simulink subsystem "lift_compoenent"  (R2024b)
settings: Solver=VariableStepAuto  StartTime=0.0  StopTime=10.0  RelTol=1e-3
values from neighbouring files (symbols this model uses):
  Ar = 0.0181458391671    [barrowaman.mat]
  Lr = 0.152    [barrowaman.mat]
  OR_cg = [-2.50212 -2.5027 -2.50328 -2.50413 -2.50497 -2.50551 -2.50605 -2.50659 -2.5076 -2.5086 -2.50952 -2.51044 ... (1300 elements, 1300x1)]    [barrowaman.mat]
  sim_time = [0.01 0.02 0.03 0.04 0.05 0.06 0.07 0.08 0.09 0.1 0.11 0.12 ... (1300 elements, 1300x1)]    [barrowaman.mat]
libraries: sharedutil x2
settings Model: Creator=joedo  LastModifiedBy=joedo

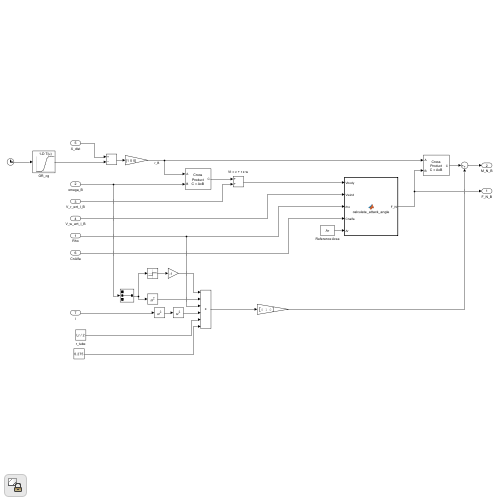
[thumbnail: Simulink's stored preview of the top-level diagram]
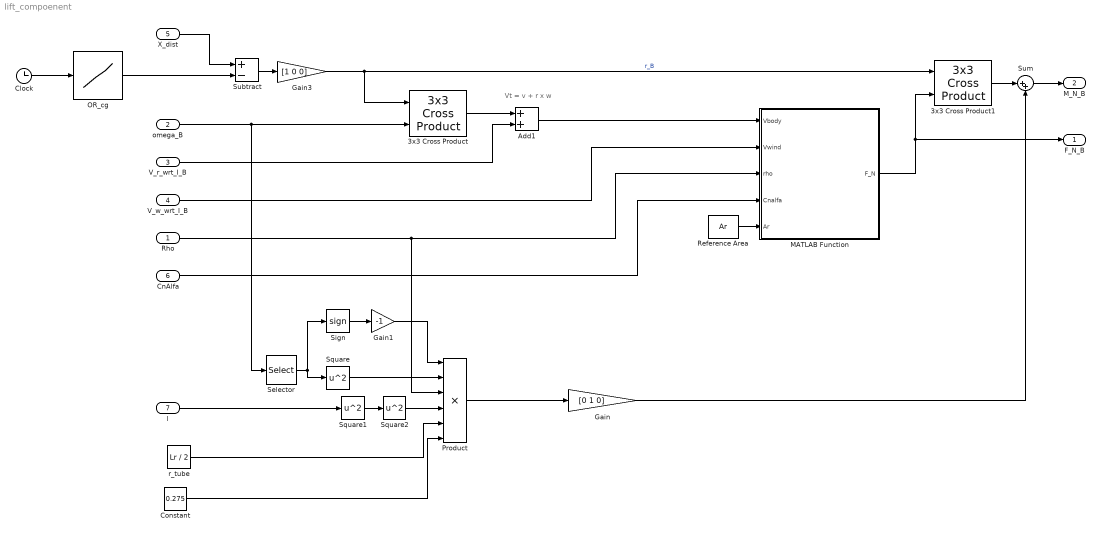
== system lift_compoenent ==
  note: Vt = v + r x w
  Rho : Inport
  omega_B : Inport  Port=2
  "V_r_wrt_I_B " : Inport  Port=3
  "V_w_wrt_I_B " : Inport  Port=4
  X_dist : Inport  Port=5
  CnAlfa : Inport  Port=6
  l : Inport  Port=7
  3x3 Cross Product : sharedutil/3x3 Cross Product  aMode=aMode
  3x3 Cross Product1 : sharedutil/3x3 Cross Product  aMode=aMode
  Add1 : Sum
  Clock : Clock
  Constant : Constant  Value=0.275
  Gain : Gain  Gain=[0 1 0]
  Gain1 : Gain  Gain=-1
  Gain3 : Gain  Gain=[1 0 0]
  MATLAB Function : MATLAB Function  TreatAsAtomicUnit=on
  OR_cg : Lookup_n-D  NumberOfTableDimensions=1  BreakpointsForDimension1=sim_time  Table=OR_cg  InternalRulePriority=Speed  RndMeth=Simplest
  Product : Product  Inputs=6
  Reference Area : Constant  Value=Ar
  Selector : Selector  InputPortWidth=3  IndexOptions=Index vector (dialog)  Indices=[2]  OutputSizes=1
  Sign : Signum
  Square : Math  Operator=square
  Square1 : Math  Operator=square
  Square2 : Math  Operator=square
  Subtract : Sum  Inputs=+-
  Sum : Sum  Inputs=|++
  r_tube : Constant  Value=Lr / 2
  F_N_B : Outport  VectorParamsAs1DForOutWhenUnconnected=off
  M_N_B : Outport  Port=2  VectorParamsAs1DForOutWhenUnconnected=off
  wires:
  omega_B/1 -> Selector/1, 3x3 Cross Product/2
  "V_r_wrt_I_B "/1 -> Add1/2
  MATLAB Function/1(F_N) -> 3x3 Cross Product1/2, F_N_B/1
  "V_w_wrt_I_B "/1 -> MATLAB Function/2(Vwind)
  3x3 Cross Product/1 -> Add1/1
  Add1/1 -> MATLAB Function/1(Vbody)
  Rho/1 -> MATLAB Function/3(rho), Product/3
  3x3 Cross Product1/1 -> Sum/1
  Gain3/1 -> 3x3 Cross Product1/1, 3x3 Cross Product/1  "r_B"
  CnAlfa/1 -> MATLAB Function/4(Cnalfa)
  Reference Area/1 -> MATLAB Function/5(Ar)
  X_dist/1 -> Subtract/1
  Subtract/1 -> Gain3/1
  Clock/1 -> OR_cg/1
  OR_cg/1 -> Subtract/2
  Selector/1 -> Square/1, Sign/1
  Square/1 -> Product/2
  l/1 -> Square1/1
  Square1/1 -> Square2/1
  r_tube/1 -> Product/5
  Square2/1 -> Product/4
  Constant/1 -> Product/6
  Product/1 -> Gain/1
  Gain/1 -> Sum/2
  Sum/1 -> M_N_B/1
  Sign/1 -> Gain1/1
  Gain1/1 -> Product/1

== matlab function lift_compoenent/MATLAB Function ==
  data: Vbody input; F_N output; Vwind input; rho input; Cnalfa input; Ar input
function F_N   = calculate_attack_angle(Vbody, Vwind, rho, Cnalfa, Ar)
%% Wind Calcs
% Body relative velocity
Vrel = Vbody - Vwind;
% Body relative velocity magnitude
Vrel_mag = norm(Vrel);
VrelMagYZ = (Vrel(3) ^ 2 + Vrel(2) ^ 2)^0.5;

%prevent division by 0
if VrelMagYZ ~= 0
    %% Angle of attack and component separation
    attack_angle = asin(VrelMagYZ/Vrel_mag);
    F_N_dir = [0, Vrel(2) / VrelMagYZ, Vrel(3) / VrelMagYZ];
    
    %% Calculating total force
    F_N_mag = (0.5 * rho * (Vrel_mag ^ 2) * Ar * Cnalfa * attack_angle);
    F_N = F_N_dir * F_N_mag;
    %F_N = F_N * 0.001;
else
    F_N = [0, 0, 0];
end
